simulink library "NoIndicators"  (R2015a)
settings: Solver=ode45  StartTime=0.0  StopTime=10.0  RelTol=1e-3
settings Model: Creator=Bruno  LastModifiedBy=Bruno

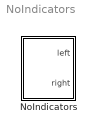
== system NoIndicators ==
  NoIndicators : Stateflow chart  TreatAsAtomicUnit=on

== stateflow chart NoIndicators/NoIndicators ==
  state Off
    entry:
    left=0; right=0
  (default) -> Off
  data: left output double size=1; right output double size=1
